simulink model "Bulker3DOFMain"  (R2023b)
settings: Solver=ode4  StartTime=0.0  StopTime=1200  FixedStep=0.01  RelTol=1e-3
libraries: simulink_extras x2, simulink x2
settings Model: Creator=myozi  LastModifiedBy=myozi

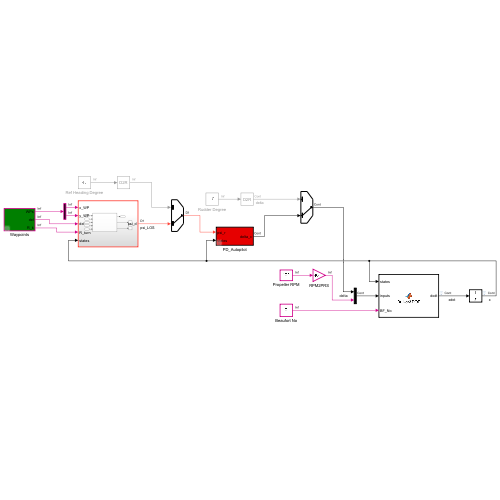
[thumbnail: Simulink's stored preview of the top-level diagram]
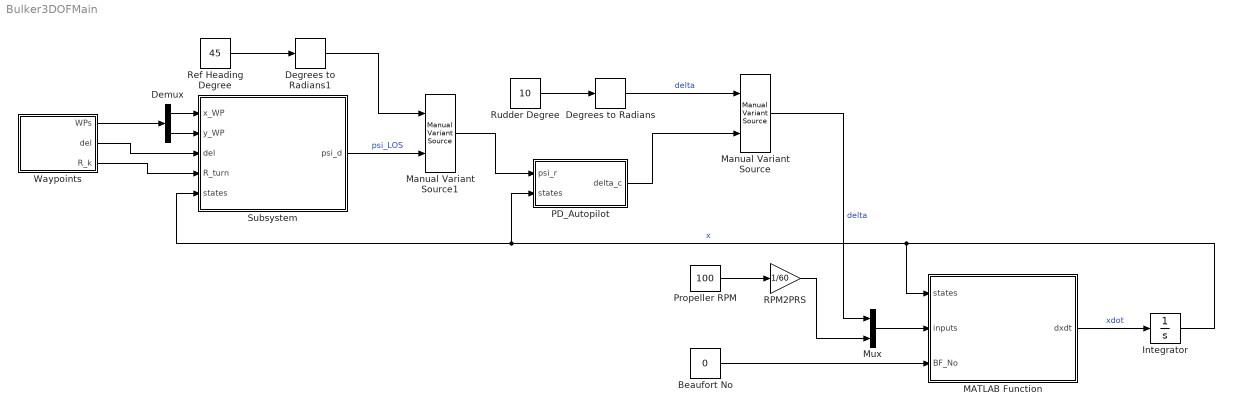
== system Bulker3DOFMain ==
  Beaufort No : Constant  Value=0
  Degrees to Radians : simulink_extras/Transformations/Degrees to Radians
  Degrees to Radians1 : simulink_extras/Transformations/Degrees to Radians
  Demux : Demux  Outputs=2
  Integrator : Integrator  InitialCondition=[0, 0, 0, 3, 0, 0]'
  MATLAB Function : MATLAB Function  TreatAsAtomicUnit=on
  Manual Variant Source : simulink/Signal Routing/Manual Variant Source  NumChoices=2  LabelModeActiveChoice=V_2
  Manual Variant Source1 : simulink/Signal Routing/Manual Variant Source  NumChoices=2  LabelModeActiveChoice=V_2
  Mux : Mux  Inputs=2
  PD_Autopilot : Subsystem  mask{K_P=3, T_D=100, T_E=1.74, delta_max=35, delta_rate=2.34}
      mask prompts: K_P "Proportional Gain :                               K_P"; T_D "Differential Time Constant : K_P*K_D = T_D"; T_E "Rudder Time Constant :                        T_E"; delta_max "Maximum Rudder Angle : delta_max (deg)"; delta_rate "Rudder Rate Limit : delta_rate (deg/s)"
      mask DialogControl Container3 Prompt: Rudder Limits
  Propeller RPM : Constant  Value=100
  RPM2PRS : Gain  Gain=1/60
  Ref Heading Degree : Constant  Value=45
  Rudder Degree : Constant  Value=10
  Subsystem : Subsystem
  Waypoints : Subsystem  mask{X_wp=[-200 1500 3000 110000 120000 300000], Y_wp=[30 -250 -1000 -70000 -90000 -300000], del=400, R_k=5*178, R_k_min=1.5*178, R_k_max=8*178}
      mask prompts: X_wp "X-Coordinates : X_wp [m]"; Y_wp "Y-Coordinates: Y_wp [m]"; del "Lookahead Distance : del (m)"; R_k "Radius of Circle of Acceptance : R_k"; R_k_min "Radius of Circle of Acceptance : R_k Minimum (m)"; R_k_max "Radius of Circle of Acceptance : R_k Max (m)"
      mask DialogControl ParameterGroupVar Prompt: Waypoints
  wires:
  MATLAB Function/1(dxdt) -> Integrator/1  "xdot"
  Integrator/1 -> Subsystem/5(states), PD_Autopilot/2(states), MATLAB Function/1(states)  "x"
  Beaufort No/1 -> MATLAB Function/3(BF_No)
  Rudder Degree/1 -> Degrees to Radians/1
  Mux/1 -> MATLAB Function/2(inputs)
  Propeller RPM/1 -> RPM2PRS/1
  Manual Variant Source/1 -> Mux/1  "delta"
  RPM2PRS/1 -> Mux/2
  PD_Autopilot/1(delta_c) -> Manual Variant Source/2
  Ref Heading Degree/1 -> Degrees to Radians1/1
  Degrees to Radians1/1 -> Manual Variant Source1/1
  Degrees to Radians/1 -> Manual Variant Source/1  "delta"
  Manual Variant Source1/1 -> PD_Autopilot/1(psi_r)
  Waypoints/1(WPs) -> Demux/1
  Waypoints/2(del) -> Subsystem/3(del)
  Subsystem/1(psi_d) -> Manual Variant Source1/2  "psi_LOS"
  Waypoints/3(R_k) -> Subsystem/4(R_turn)
  Demux/1 -> Subsystem/1(x_WP)
  Demux/2 -> Subsystem/2(y_WP)

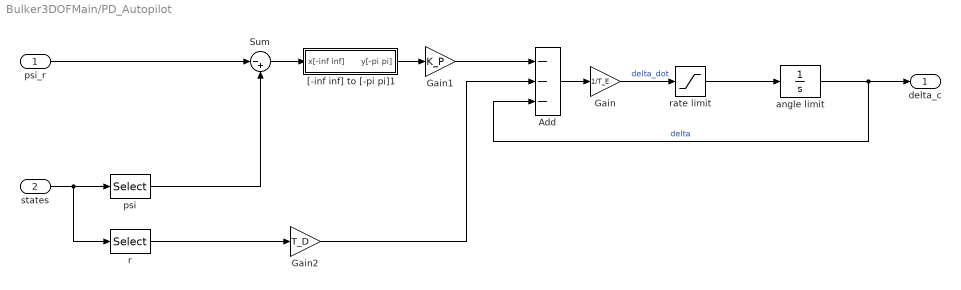
== system Bulker3DOFMain/PD_Autopilot ==
  psi_r : Inport
  states : Inport  Port=2
  Add : Sum  Inputs=---
  Gain : Gain  Gain=1/T_E
  Gain1 : Gain  Gain=K_P
  Gain2 : Gain  Gain=T_D
  Sum : Sum  Inputs=|-+
  "[-inf inf] to [-pi pi]1" : Subsystem
  angle limit : Integrator  LimitOutput=on  UpperSaturationLimit=delta_max*pi/180  LowerSaturationLimit=-delta_max*pi/180
  psi : Selector  InputPortWidth=6  IndexOptions=Index vector (dialog)  Indices=[3]  OutputSizes=1
  r : Selector  InputPortWidth=6  IndexOptions=Index vector (dialog)  Indices=[6]  OutputSizes=1
  rate limit : Saturate  UpperLimit=delta_rate*pi/180  LowerLimit=-delta_rate*pi/180
  delta_c : Outport  VectorParamsAs1DForOutWhenUnconnected=off
  wires:
  psi_r/1 -> Sum/1
  Add/1 -> Gain/1
  Gain1/1 -> Add/1
  Sum/1 -> "[-inf inf] to [-pi pi]1"/1(x[-inf inf])
  Gain/1 -> rate limit/1  "delta_dot"
  angle limit/1 -> Add/3, delta_c/1  "delta"
  Gain2/1 -> Add/2
  "[-inf inf] to [-pi pi]1"/1(y[-pi pi]) -> Gain1/1
  states/1 -> r/1, psi/1
  rate limit/1 -> angle limit/1
  psi/1 -> Sum/2
  r/1 -> Gain2/1

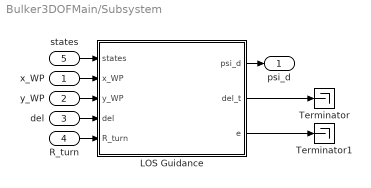
== system Bulker3DOFMain/Subsystem ==
  x_WP : Inport
  y_WP : Inport  Port=2
  del : Inport  Port=3
  R_turn : Inport  Port=4
  states : Inport  Port=5
  LOS Guidance : MATLAB Function  TreatAsAtomicUnit=on  VariantControl=varient3
  Terminator : Terminator
  Terminator1 : Terminator
  psi_d : Outport
  wires:
  states/1 -> LOS Guidance/1(states)
  x_WP/1 -> LOS Guidance/2(x_WP)
  del/1 -> LOS Guidance/4(del)
  LOS Guidance/2(del_t) -> Terminator/1
  LOS Guidance/1(psi_d) -> psi_d/1
  y_WP/1 -> LOS Guidance/3(y_WP)
  LOS Guidance/3(e) -> Terminator1/1
  R_turn/1 -> LOS Guidance/5(R_turn)

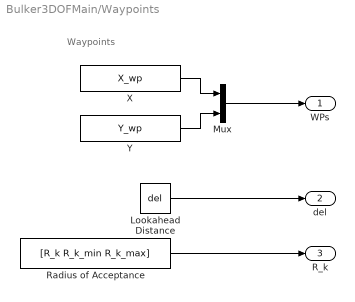
== system Bulker3DOFMain/Waypoints ==
  note: Waypoints
  Lookahead Distance : Constant  Value=del
  Mux : Mux  Inputs=2
  Radius of Acceptance : Constant  Value=[R_k R_k_min R_k_max]
  X : Constant  Value=X_wp
  Y : Constant  Value=Y_wp
  WPs : Outport  VectorParamsAs1DForOutWhenUnconnected=off
  del : Outport  Port=2  VectorParamsAs1DForOutWhenUnconnected=off
  R_k : Outport  Port=3  VectorParamsAs1DForOutWhenUnconnected=off
  wires:
  Y/1 -> Mux/2
  X/1 -> Mux/1
  Radius of Acceptance/1 -> R_k/1
  Lookahead Distance/1 -> del/1
  Mux/1 -> WPs/1

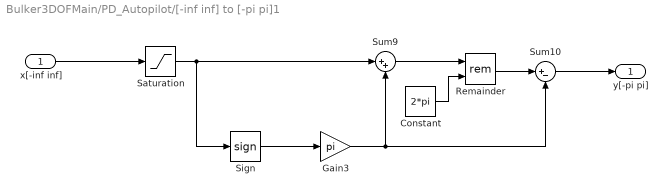
== system Bulker3DOFMain/PD_Autopilot/[-inf inf] to [-pi pi]1 ==
  x[-inf inf] : Inport
  Constant : Constant  Value=2*pi
  Gain3 : Gain  Gain=pi
  Remainder : Math  Operator=rem  SignedPower=on
  Saturation : Saturate  UpperLimit=1e10  LowerLimit=-1e10
  Sign : Signum
  Sum10 : Sum  Inputs=|+-
  Sum9 : Sum  Inputs=|++
  y[-pi pi] : Outport  VectorParamsAs1DForOutWhenUnconnected=off
  wires:
  Sum9/1 -> Remainder/1
  x[-inf inf]/1 -> Saturation/1
  Remainder/1 -> Sum10/1
  Sum10/1 -> y[-pi pi]/1
  Sign/1 -> Gain3/1
  Saturation/1 -> Sum9/1, Sign/1
  Gain3/1 -> Sum9/2, Sum10/2
  Constant/1 -> Remainder/2

== matlab function Bulker3DOFMain/MATLAB Function ==
  data: states input; dxdt output; inputs input; BF_No input
function dxdt = Bulker3DOF(states,inputs,BF_No)

dxdt = Bulker3DOF(states,inputs,BF_No);

== matlab function Bulker3DOFMain/Subsystem/LOS Guidance ==
  settings: updateMethod=DISCRETE
  data: states input; x_WP input; y_WP input; del input; R_turn input; psi_d output; del_t output; e output
function [psi_d, del_t, e]  = LOSStraight(states,x_WP,y_WP,del,R_turn)

[psi_d, del_t, e]   = LOSStraight(states,x_WP,y_WP,del,R_turn);
